simulink library "snn_champions_lib"  (R2026a)
settings: Solver=VariableStepAuto
(part 11 of 24)

== matlab function snn_champions_lib/Donatello_Tier/VS/SLOW_n8/DEC ==
  data: raw input; v0 output; valid input; T output; s0 output; a output; b output
function [v0, T, s0, a, b] = DEC(raw, valid)
%#codegen
% [SPLIT] Solo il decode: latch di raw + fasi. Riceve raw(5)+valid dalla MF SNN (entita' a se').
  persistent pv rawl dodec
  if isempty(pv)
    pv = fi(zeros(5,1), 1, 21, 13);
    rawl = fi(zeros(5,1), 1, 21, 13);
    dodec = false;
  end
  if dodec
    pv = snn_decode_lut(rawl, 64);
    dodec = false;
  end
  if valid
    rawl(:) = raw;               % latch DOPO la catena: rawl e' un vero registro
    dodec = true;
  end
  v0 = pv(1); T = pv(2); s0 = pv(3); a = pv(4); b = pv(5);
end

% ====================================================================================
% Funzioni locali INLINATE dai sorgenti veri (build_hdl_variants le legge a build-time).
% Le funzioni locali hanno precedenza sul path => il blocco e' SELF-CONTAINED.
% NON modificarle qui: si rigenerano con build_hdl_variants.
% ====================================================================================

function p = snn_decode_lut(raw, N) %#codegen
%SNN_DECODE_LUT  Decode Donatello con sigmoide via LUT a N punti su [-8,8) + interp lineare.
%  Generalizza snn_decode_hdl (N=256). N = coder.const, potenza di 2 (scala indice = N/16).
%  Costanti Donatello baked (lo sweep e' Donatello-only). Bit-identico a snn_decode_hdl per N=256.
%
%  ⚠️ SINGLE SOURCE (R4, 2026-07-19): il corpo e' ora la composizione di decode_a + decode_b, che sono
%  le DUE FASI che la chart esegue in due clock distinti -- il decode era il collo (pv_3, 31 livelli:
%  quattro moltiplicatori in serie piu' la lettura di tabella, tutto in un clock).
%  Composte qui in una chiamata sola perche' (a) i chiamanti non cambiano (snn_top_b2, le varianti
%  Donatello_LUT16..512) e (b) i cancelli provano ESATTAMENTE il codice che gira in hardware, non un
%  suo gemello. Il taglio e' fra `frac` e la lettura di `sgtab`: espressioni invariate, solo separate.
  [k, frac] = decode_a(raw, N);
  sv        = decode_b(k, frac, N);
  p         = decode_c(sv);   % [R10] scalatura finale in una fase a se'
end


function [k, frac] = decode_a(raw, N) %#codegen
%DECODE_A  [R4/R12] Prima meta' del decode: dal readout grezzo all'INDICE di tabella + frazione.
%
%  ⚠️ SINGLE SOURCE: composizione di decode_a1 (normalizzazione) e decode_a2 (scala/indice/frazione),
%  che la chart esegue in DUE clock -- i due moltiplicatori erano in serie (collo a 57,5 MHz).
%  Composta qui per i chiamanti funzionali (snn_decode_lut) e perche' i cancelli provino il codice vero.
%
%  ⚠️ NON si time-multiplexano i 5 parametri (restano srotolati): sarebbe un'ottimizzazione di AREA, e
%  di area ce n'e' in abbondanza. Serve solo profondita'.
  adjv        = decode_a1(raw);
  [k, frac]   = decode_a2(adjv, N);
end


function adjv = decode_a1(raw) %#codegen
%DECODE_A1  [R12] Prima parte del decode: normalizzazione (raw - offset)*invtau.
%  Separata da decode_a2 perche' i due moltiplicatori (invtau e scale) erano in serie nello stesso
%  clock -- era il collo a 57,5 MHz (dfrv, 18 livelli). `adj` ha il tipo Tadj GIA' DICHIARATO
%  nell'originale, quindi qui non si stringe nulla (nessun rischio §2.1).
%  Espressione VERBATIM da snn_decode_lut.
  Traw  = numerictype(1,21,13); Tadj = numerictype(1,18,13); Titau = numerictype(1,18,16);
  offset = coder.const(fi([-0.40404 -0.39012 1.7718 2.6884 -0.95578].', Traw));
  invtau = coder.const(fi([0.1 1/3 0.1 1/3 1/3].', Titau));
  adjv = fi(zeros(5,1), Tadj);
  for i = 1:5
    adjv(i) = fi((raw(i) - offset(i)) * invtau(i), Tadj);
  end
end


function [k, frac] = decode_a2(adjv, N) %#codegen
%DECODE_A2  [R12] Seconda parte: scala su [0,N), indice di tabella e frazione.
%  Espressioni VERBATIM da snn_decode_lut, con `adj` gia' calcolato da decode_a1.
  Tadj = numerictype(1,18,13); Ts = numerictype(1,16,14); Tsc = numerictype(0,23,13);
  scale = coder.const(N / 16);                                    % punti per unita' su [-8,8)
  Tsm   = numerictype(0, 8, 0);                                   % moltiplicatore scala (<=32)
  k    = zeros(5, 1, 'int32');
  frac = fi(zeros(5,1), Ts);
  for i = 1:5
    scaled = fi((adjv(i) + fi(8, Tadj)) * fi(scale, Tsm), Tsc);    % (adj+8)*scale in [0,N)
    ki = int32(floor(scaled));
    if ki < int32(0),     ki = int32(0);     end
    if ki > int32(N - 2), ki = int32(N - 2); end
    k(i)    = ki;
    frac(i) = fi(scaled - fi(double(ki), Tsc), Ts);
  end
end


function sv = decode_b(k, frac, N) %#codegen
%DECODE_B  [R4/R10/R17] Seconda fase del decode: tabella + interpolazione lineare -> s.
%  ⚠️ SINGLE SOURCE: composizione di decode_b1 (letture + differenza) e decode_b2 (interpolazione), che
%  la chart esegue in DUE clock. Composta qui per i chiamanti funzionali e per i cancelli.
  [s0v, delv] = decode_b1(k, N);
  sv          = decode_b2(s0v, delv, frac);
end


function [s0v, delv] = decode_b1(k, N) %#codegen
%DECODE_B1  [R17] Letture della tabella + differenza: s0 = sgtab(k), del = sgtab(k+1) - sgtab(k).
%  Separata da decode_b2 perche' letture, sottrazione, moltiplicazione e somma erano tutte nello stesso
%  clock -- era il collo a 77,6 MHz (dsv, 14 livelli). Espressioni VERBATIM da snn_decode_lut.
  Ts    = numerictype(1,16,14);
  scale = coder.const(N / 16);
  sgtab = coder.const(fi(1 ./ (1 + exp(-(-8 + (0:N-1) / scale))), Ts));  % 1xN
  s0v  = fi(zeros(5,1), Ts);
  delv = fi(zeros(5,1), Ts);
  for i = 1:5
    s0 = sgtab(k(i) + 1); s1 = sgtab(k(i) + 2);
    s0v(i)  = s0;
    delv(i) = fi(s1 - s0, Ts);
  end
end


function sv = decode_b2(s0v, delv, frac) %#codegen
%DECODE_B2  [R17] Interpolazione lineare: s = s0 + frac*del. Espressione VERBATIM da snn_decode_lut.
  Ts = numerictype(1,16,14);
  sv = fi(zeros(5,1), Ts);
  for i = 1:5
    sv(i) = fi(s0v(i) + frac(i) * delv(i), Ts);
  end
end


function p = decode_c(sv) %#codegen
%DECODE_C  Scalatura finale -> i 5 parametri. [R10] fase a se' nel controllore.
%  [A3] Ora e' la COMPOSIZIONE di decode_c1 (i prodotti, a precisione piena) + decode_c2 (somma
%  dell'offset + cast). Composta qui perche' (a) i chiamanti non cambiano e (b) i cancelli provano
%  ESATTAMENTE il codice che gira in hardware, non un suo gemello.
%  La chart nella variante `p6` chiama le due meta' in due fasi distinte: e' li' che il taglio serve,
%  perche' separa i DSP dalla catena di CARRY4 che domina il path critico.
  pr = decode_c1(sv);
  p  = decode_c2(pr);
end


function pr = decode_c1(sv) %#codegen
%DECODE_C1  [A3] Prima meta' di decode_c: i SOLI PRODOTTI hilo.*sv.
%  Taglio dentro l'operazione, non fra le operazioni: il collo di Donatello e' `lo + hilo*sv`, dove i
%  DSP fanno la moltiplicazione ma la somma finisce in fabric come catena di 15 CARRY4 in serie
%  (misurato: 24,307 ns = logica 15,490 + routing 8,817, 23 livelli).
%  Registrare il prodotto separa DSP e addizionatore in due clock.
%
%  ⚠️ LARGHEZZA PIENA: il prodotto NON va stretto qui. Stringere un parziale prima dell'uso e' il bug
%  §2.1 di questo progetto — cambierebbe la matematica. Il tipo si lascia DEDURRE dall'espressione.
  Tp   = numerictype(1,21,13);
  hilo = coder.const(fi([37 2 4 2.2 2.5].', Tp));
  pr   = hilo .* sv;                  % tipo dedotto = precisione piena
end


function p = decode_c2(pr) %#codegen
%DECODE_C2  [A3] Seconda meta' di decode_c: somma dell'offset + cast finale ai 5 parametri.
%  Riceve il prodotto a PRECISIONE PIENA da decode_c1 (registrato) e fa `lo + pr`, poi il cast a Q8.13.
%  Aritmetica IDENTICA a decode_c: stesso ordine, stesso singolo cast finale -> bit-exact per
%  costruzione. Ma "per costruzione" non e' un cancello: lo prova run_block_traj_test (dmax=0).
  Tp = numerictype(1,21,13);
  lo = coder.const(fi([8 0.5 1 0.3 0.5].', Tp));
  p  = fi(zeros(5,1), Tp);
  for i = 1:5
    p(i) = fi(lo(i) + pr(i), Tp);
  end
end

== matlab function snn_champions_lib/Leonardo/SNN ==
  data: x_phys input; params output
function params = SNN(x_phys)
%#codegen
% Blocco champion SELF-CONTAINED: pesi bakati + forward ALIF + decode, zero dipendenze .m.
  W_IN  = [0.25 1 0 0.5;-0.25 0.125 -1 1;0.125 -0.5 1 0.5;1 0.25 0.5 -0.25;1 0.25 -0.25 0.125;-0.25 0.5 -0.5 1;-1 -0.5 -0.5 -1;-0.0625 -1 1 -1;0.5 0.125 -0.5 0.5;-0.125 1 0.25 -0.5;-0.125 -0.125 0.5 1;0.5 -0.0625 1 0;1 -0.5 -0.5 0.5;-1 1 0.25 0.0625;0.25 -0.25 1 -1;0 -0.5 0.25 -0.125;0.5 -0.125 1 -0.5;-1 -1 0.5 0.0625;1 -0.5 -1 -0.5;-1 0.5 0.25 1;-1 -1 1 0;0.5 -0.5 0.25 -1;-0.5 0.5 0.25 -0.25;0.5 1 -0.5 -0.25;0.5 -0.25 -0.5 -1;-0.5 0.25 -0.5 -0.5;0.25 -0.5 -1 -0.25;-2 -0.5 1 0.0625;0.5 -1 -1 -1;0.125 -1 0.125 0.5;0.5 -0.5 -0.25 -0.5;-0.5 -0.25 -0.25 0.5];
  U     = [-0.25 0.0625 -0.125 -0.125 -0.25 0.0625 0.25 0.0625;-0.0625 -0.125 0.125 0.0625 -0.125 -0.0625 0 -0.0625;-0.125 -0.0625 -0.125 -0.0625 -0.0625 0 0.125 0;0.125 0.0625 0.125 0.125 -0.0625 0.0625 -0.25 0;0.125 0.0625 0.125 0.25 0.125 -0.0625 0 -0.0625;0.25 -0.125 0.25 0.25 0 -0.125 -0.25 -0.25;0.25 -0.25 0.5 0.0625 0.25 -0.25 -0.5 -0.5;0.25 -0.125 0.25 0.125 0.125 -0.125 -0.25 -0.25;0.125 -0.125 0.25 0 0.5 -0.25 -0.25 -0.125;-0.125 0.25 -0.25 0 -0.125 0.25 0.25 0.25;-0.25 0.0625 -0.25 -0.125 -0.25 0 0.25 0.125;-0.125 0.25 -0.125 -0.125 0 0.0625 0.25 0.125;0.125 0.125 0.0625 0.25 0.25 0.125 0 -0.0625;0.0625 0 0.0625 0.125 -0.25 0.125 0 0.125;-0.25 0.125 -0.0625 -0.25 0.125 0.0625 0.125 0.125;-0.125 -0.0625 -0.125 0.125 -0.25 -0.125 0.0625 0;0.5 -0.25 0.25 -0.0625 0.5 -0.5 -0.5 -0.25;0.125 -0.25 0.125 0.125 0.25 -0.25 -0.25 -0.0625;0.25 -0.25 0.25 0.0625 0.125 -0.25 -0.25 -0.25;-0.0625 -0.125 0 0.125 -0.25 0 0.125 0.0625;-0.25 0.125 -0.25 -0.125 -0.0625 0.125 0.25 0.25;0.25 -0.25 0.25 0.125 0.25 -0.25 -0.25 -0.25;0.125 -0.0625 0.0625 0.5 0.0625 0.25 0 0;0.125 -0.25 0.25 0.5 0.125 -0.125 0 -0.25;-0.25 -0.0625 -0.0625 0 -0.0625 0 0.25 0;0.5 -0.25 0.25 0.25 0.25 -0.5 -0.25 -0.25;0.5 -0.5 0.5 0.5 0.25 -0.25 -0.5 -0.5;0.125 -0.25 0.25 0.125 0.25 -0.0625 0.0625 -0.125;0.5 -0.25 0.5 0.0625 0.5 -0.5 -0.5 -0.5;-0.25 0.25 -0.5 -0.25 -0.25 0.25 0.5 0.5;0.5 -0.5 0.5 0.125 0.5 -0.5 -0.5 -0.25;0 -0.0625 0.125 -0.0625 0.0625 -0.125 -0.125 -0.0625];
  V     = [0.0625 -0.25 -0.125 0.25 0.25 0.125 0 -0.125 -0.25 0.25 -0.125 -0.0625 0 0.125 -0.125 0.0625 -0.125 -0.25 -0.25 -0.125 -0.25 -0.25 1 0.25 0.25 -0.0625 -0.0625 -0.25 0 0 -0.125 0;-0.125 -0.125 -0.0625 0 0 -0.125 0 0.125 0.5 -0.125 0 0.0625 -0.125 -0.125 -0.125 0.125 0.25 0.25 -0.25 -0.25 0 -0.25 -0.25 0 -0.25 -0.125 -0.0625 0.0625 0 0 0.125 0;0.125 0.0625 0 0.0625 0 0.5 0 0 -0.0625 0.125 0 -0.0625 0.25 0.125 0 0 -0.125 -0.25 0.25 0.125 -0.25 -0.25 0.5 0.125 0.125 -0.125 0.0625 -0.125 0 -0.0625 -0.125 0;0 -0.125 -0.125 0.0625 -0.0625 0 0.0625 -0.25 -0.25 0.25 -0.125 -0.125 0.125 0.125 -0.125 0.0625 -0.25 -0.25 -0.5 0.0625 -0.25 -0.5 1 0.125 0.0625 0 -0.125 0.0625 0 0 -0.25 0;0.0625 -0.5 0.0625 0.125 -0.0625 0 -0.0625 -0.25 -0.125 0.25 -0.0625 0.25 0.0625 0.0625 -0.25 -0.0625 0.0625 -0.25 -0.0625 -0.125 -0.25 -0.25 0.0625 0.125 0 -0.25 -0.125 -0.125 -0.0625 -0.125 0 -0.0625;-0.125 -0.125 -0.0625 -0.125 0 -0.25 0 0 0.25 0 -0.125 -0.125 0.25 -0.0625 -0.125 0 0.0625 0.25 -0.5 -0.0625 0.25 0.125 0 0.125 -0.25 0.125 -0.125 0.25 -0.0625 0.125 0.25 0;-0.25 0.0625 0.0625 -0.25 -0.25 -0.25 -0.0625 -0.0625 0.0625 -0.0625 -0.0625 -0.125 0 0.0625 -0.125 -0.0625 -0.0625 0.25 -0.25 0.125 0.25 0 -0.125 -0.0625 -0.25 0.25 -0.125 0.5 0 0.0625 0.125 0;-0.125 0.125 0 -0.125 0 -0.25 0 0.125 0.125 -0.0625 -0.0625 0 0.0625 -0.125 -0.0625 -0.0625 0 0.25 -0.5 -0.0625 0.25 0.0625 -0.5 0.0625 -0.125 0.0625 0 0.25 0 0.125 0.25 0.0625];
  DEL   = [3 5 1 2;2 4 4 4;2 4 0 4;5 0 5 5;1 2 2 2;4 1 4 2;0 4 0 1;0 1 0 1;2 2 1 3;1 2 5 2;0 5 1 2;0 5 3 1;2 0 0 4;2 2 3 4;4 4 5 0;4 5 0 2;0 4 4 3;5 5 4 2;4 5 4 2;3 0 3 1;3 2 0 4;0 4 2 0;5 4 5 2;4 4 3 3;5 3 4 5;2 2 3 1;3 3 5 3;1 3 0 3;1 0 3 2;2 3 4 4;2 4 5 0;1 2 4 0];
  BTH   = [1.5400424003601074;0.60637873411178589;1.2149713039398193;1.3223150968551636;1.5843478441238403;1.3005355596542358;1.4105348587036133;1.0825026035308838;1.3853039741516113;1.0379821062088013;1.2504197359085083;1.158677339553833;0.93588978052139282;1.1027405261993408;1.3031506538391113;1.3676879405975342;1.6325922012329102;1.5050898790359497;1.0741523504257202;1.2025256156921387;1.0485290288925171;1.5150537490844727;0.84104228019714355;0.99839270114898682;1.5752084255218506;1.2629411220550537;1.3518692255020142;0.76825004816055298;1.4178869724273682;1.114804744720459;1.1964786052703857;1.3985182046890259];
  TJ    = [0.53961282968521118;-0.065692238509654999;0.69547575712203979;0.39467334747314453;0.27812755107879639;0.36636638641357422;0.46853935718536377;0.28439891338348389;0.26325023174285889;0.12272599339485168;0.57048964500427246;0.35351014137268066;-0.00250800303183496;-0.027677660807967186;0.63428056240081787;0.40770524740219116;0.74491316080093384;0.59902232885360718;0.20256176590919495;-0.0053168567828834057;0.3602060079574585;0.55292367935180664;-0.0063420552760362625;-0.055277645587921143;0.62946045398712158;0.42266586422920227;0.35328882932662964;-0.024216080084443092;0.47340747714042664;0.37444651126861572;0.26409748196601868;0.46853935718536377];
  LD    = [8;8;8;8;8;8;8;8;8;8;8;8;8;8;8;8;8;8;8;8;8;8;8;8;8;8;8;8;8;8;8;8];
  W_OUT = [0.125 2 0 0.125 0.0625 0.5 -0.0625 0.5 0.125 -0.125 0.25 -0.25 0.125 0.5 0 1 -0.5 -0.25 0.5 1 0.25 1 -0.125 0.5 0.25 0.25 0.5 -2 -0.25 1 -0.5 0.5;-0.125 -0.25 -0.25 0.125 0.25 0.0625 0 0.25 0.25 -0.125 -0.25 0.0625 0.5 -0.25 -0.0625 0.25 0.25 0.0625 -0.125 -0.125 0 0.5 -0.25 0.0625 -0.5 -0.25 0.125 -0.5 0.125 0.25 0.0625 -0.0625;-0.5 -0.25 -0.5 -0.125 0.5 0.5 0.125 -0.5 0.125 -1 -1 -1 0.5 -0.5 -0.25 -0.25 -0.0625 0.0625 0.0625 -0.5 -1 -0.0625 -0.125 0.5 0.125 0 0.5 -0.125 0.125 -0.5 0.25 -0.125;-0.25 0.25 0.0625 -0.25 -0.125 -0.125 -0.125 0.125 -0.125 -0.5 -0.125 -0.25 0.0625 -0.5 0.25 -0.125 -0.0625 -0.25 0.25 -0.0625 0.125 0.5 -1 -0.5 -0.0625 -0.25 0 -0.5 -0.125 0.125 0.25 0.0625;-0.125 -0.5 -0.25 -0.0625 0.125 0.25 0.25 -0.125 0.5 -0.0625 -0.25 -0.0625 1 -0.25 -0.25 0.0625 0.125 -0.0625 0.5 -0.25 -0.25 0 -0.125 0.125 -0.125 0 -0.25 -0.25 0.25 -1 -0.125 0.25];
  P_LO  = [8;0.5;1;0.30000001192092896;0.5];
  P_HI  = [45;2.5;5;2.5;3];
  D_OFF = [-0.67073744535446167;-0.11699806153774261;-1.4559782743453979;-0.27981284260749817;-1.7696963548660278];
  L_TAU = [10;3;10;3;3];
  NRM   = [150;40;20;40];
  NT = 10; MAXD = 6; H = size(W_IN, 1);
  % --- normalizzazione (fisico -> [0,1]) ---
  xin = x_phys(:);
  dvc = min(max(xin(3), -NRM(3)), NRM(3));
  xn  = [xin(1)/NRM(1); xin(2)/NRM(2); (dvc + NRM(3))/(2*NRM(3)); xin(4)/NRM(4)];
  % --- stato persistente (registri del blocco) ---
  persistent Vm fat sprev Vli xbuf started
  if isempty(started)
    Vm = zeros(H,1); fat = zeros(H,1); sprev = zeros(H,1);
    Vli = zeros(5,1); xbuf = zeros(4, MAXD); started = true;
  end
  % --- NT tick SNN interni ---
  for k = 1:NT
    xbuf(:, 2:end) = xbuf(:, 1:end-1); xbuf(:, 1) = xn;
    Iin = zeros(H, 1);
    for dd = 0:MAXD-1
      mask = double(DEL == dd);
      Iin = Iin + (W_IN .* mask) * xbuf(:, dd+1);
    end
    rec = U * (V * sprev);
    Vm  = Vm - Vm ./ LD + Iin + rec;
    eth = BTH + max(fat, 0);
    s   = double(Vm >= eth);
    fat = fat - fat ./ LD + s .* max(TJ, 0);
    Vm  = Vm - s .* eth;
    sprev = s;
    Vli = Vli - Vli ./ 8 + W_OUT * s;
  end
  % --- decode -> 5 parametri fisici ---
  adj = (Vli - D_OFF) ./ L_TAU;
  params = P_LO + (P_HI - P_LO) .* (1 ./ (1 + exp(-adj)));
end

== matlab function snn_champions_lib/Donatello_Tier/VS/SLOW_n5/SNN ==
  data: s input; raw output; v input; dv input; v_l input; valid output
function [raw, valid] = SNN(s, v, dv, v_l)
%#codegen
% [SPLITPIPE] REGISTRO sugli OPERANDI del normalize (fra clamp e moltiplicazione): la
% moltiplicazione a 34 bit finisce in uno stadio suo -> rompe ingresso->normalize->go. La
% moltiplicazione e' a valle di op_reg; l'edge-trigger confronta gli OPERANDI registrati (equivale
% a confrontare xn, dato che mul e' deterministica). +1 clock di latenza. Fuori dal core.
  Tt = snn_types('fixed', 5);
  op = local_normalize_ops(s, v, dv, v_l);
  persistent op_reg op_prev started prime
  if isempty(started)
    op_reg = cast(zeros(4,1), 'like', op);  % init COSTANTE (non =op: eviterebbe il registro
    op_prev = op_reg;                        %  con un bypass combinatorio ingresso->mul->xbuf)
    started = true; prime = true;
    go = false;
  elseif prime
    prime = false;
    go = true;
  else
    go = any(op_reg ~= op_prev);
  end
  op_prev = op_reg;
  xn = local_normalize_mul(op_reg, Tt);
  [raw, valid] = snn_b2_fsm(xn, go);
  op_reg = op;
end

function xn = local_normalize(s, v, dv, v_l, T)
%LOCAL_NORMALIZE  fisico -> xn (fixed) = composizione ops+mul (bit-identica all'originale).
%  Nel deployato la normalize gira in SW float e all'HDL arriva gia' xn (HDL_PHASE §3.1).
  op = local_normalize_ops(s, v, dv, v_l);
  xn = local_normalize_mul(op, T);
end

function op = local_normalize_ops(s, v, dv, v_l)
%LOCAL_NORMALIZE_OPS  clamp del dv -> operandi [s; v; d_clamped; v_l] (pre-moltiplicazione).
  DVc = fi(20, 1, 24, 13);   % 24-13-1 = 10 bit interi: DV=20 ci sta
                                   % (con Q5.13/18bit saturerebbe a ~16 -> clamp sbagliato)
  d = dv;                          % clamp a +-DV. NB: d(:) = ... per NON cambiare il tipo di d
  if d >  DVc, d(:) =  DVc; end    %     (codegen: una variabile non puo' cambiare tipo, HDL_PHASE §9)
  if d < -DVc, d(:) = -DVc; end
  op = [s; v; d; v_l];
end

function xn = local_normalize_mul(op, T)
%LOCAL_NORMALIZE_MUL  operandi -> xn. RECIPROCI a Q?.30 (NON Q?.20): con Q?.20 xn devia di 1 LSB
%  ~1 volta su 25 step -> uno spike flippa -> params divergono. Con Q?.30 e ingressi >=20 bit
%  frazionari, xn e' IDENTICO al riferimento float (0 diff).
  invS   = fi(0.0066666666666666671, 1, 34, 30);
  invV   = fi(0.025000000000000001, 1, 34, 30);
  inv2DV = fi(0.025000000000000001, 1, 34, 30);
  invVL  = fi(0.025000000000000001, 1, 34, 30);
  DVc    = fi(20, 1, 24, 13);
  xn = cast(zeros(4,1), 'like', T.V);
  xn(1) = cast(op(1) * invS, 'like', T.V);
  xn(2) = cast(op(2) * invV, 'like', T.V);
  xn(3) = cast((op(3) + DVc) * inv2DV, 'like', T.V);
  xn(4) = cast(op(4) * invVL, 'like', T.V);
end

% ====================================================================================
% Funzioni locali INLINATE dai sorgenti veri (build_hdl_variants le legge a build-time).
% Le funzioni locali hanno precedenza sul path => il blocco e' SELF-CONTAINED.
% NON modificarle qui: si rigenerano con build_hdl_variants.
% ====================================================================================

function W = b2_rom_active() %#codegen
%B2_ROM_ACTIVE  Pesi del champion attivo (baked). GENERATO da gen_b2_rom('Donatello').
  W.fc = fi([1 1 -0.25 1;0.125 0.5 -0.0625 1;1 -1 1 0.125;1 0.125 0.5 -0.125;1 0.5 -0.0625 0.5;-0.0625 0.25 0 1;0 0.5 0.5 0.25;1 -0.25 2 -0.0625;1 0.125 -0.25 0.5;0.25 1 0.125 -0.25;0.25 -0.25 0.5 1;0.5 -0.5 0.5 0.25;1 0.25 -0.125 0.5;-1 1 0.25 0.5;1 0.5 1 -0.25;0.5 -0.25 0.5 0.0625;0.25 -0.25 1 -0.5;-0.5 -0.5 1 0.25;2 0 -0.25 0;-0.5 0.5 0.5 1;-0.125 -0.25 1 0;1 0.125 1 -0.5;-0.0625 1 0.5 0.125;1 1 -0.25 -0.125;2 0.5 0.5 -0.25;-0.125 0.5 0.25 -0.25;1 0.125 -0.0625 0.25;-0.5 -0.25 1 0.5;1 -0.125 0.125 0.5;1 -0.0625 0.5 0.25;1 0.5 1 0.125;0.125 0.25 0.5 0], 1, 16, 13);
  W.U = fi([0 0 -0.0625 -0.0625 -0.0625 0 0 0 -0.0625 0 0 0 0.0625 0 -0.125 0;-0.0625 0 -0.0625 0 0 0 0 0 0 0 -0.0625 0 0 0.0625 0 0;0.0625 -0.0625 -0.0625 0 -0.0625 -0.0625 0 0 0.0625 0 0.0625 0 0 0 0 0;0.0625 -0.0625 0 0 0 0 -0.0625 0 0 -0.0625 0.0625 -0.0625 0 -0.0625 0 -0.0625;0.0625 -0.0625 0 0 0 0 0.0625 0 0 0 0 -0.0625 0.0625 0 -0.0625 0;0 0.0625 0.0625 -0.0625 0.0625 0 0 0 0.0625 0.0625 0 0.0625 0 0 0 0;-0.0625 0.0625 0.0625 -0.0625 0 0 -0.0625 0.0625 0.0625 0.0625 0 0 -0.0625 0 0 0.0625;0 0 0.0625 0.0625 0 0 0 0 -0.0625 -0.0625 0 0 0 0 -0.0625 0;0 0 0 0 0.0625 -0.0625 0 0 -0.0625 -0.0625 -0.0625 0 0 0 0.0625 0;0 0 0 0 0.0625 0 0 0 0.0625 -0.0625 0 0.0625 0 0 0 0.0625;0 0 0 0 0 0 0 -0.0625 0 0 -0.0625 0 0 0 0 0.0625;0 0.0625 0 0.0625 0 0 0 0.0625 0 -0.0625 0 -0.0625 0.0625 0 0 0;-0.0625 0.0625 0 0 0 0 -0.0625 0 0.0625 0 -0.0625 0 0 0 0 0.125;0 0 0 0 0 0.0625 -0.0625 -0.0625 0 0.0625 0 0 0.0625 0.0625 0.0625 0;0.0625 0.0625 -0.0625 0 0 -0.0625 -0.0625 0 0 0 -0.0625 0 -0.0625 0 0 0;0.0625 0 0 0 -0.0625 -0.0625 -0.0625 0.0625 -0.0625 -0.0625 0 0.0625 0 0 0 0.0625;-0.0625 0 0 0 0.125 0.0625 -0.0625 -0.0625 0 0 0 0 -0.0625 0 -0.0625 0;0.0625 -0.0625 0 0.0625 0 -0.125 0 -0.0625 0 0 0.0625 -0.0625 0.0625 0 -0.0625 -0.0625;-0.0625 0 -0.0625 0.0625 -0.0625 0 -0.0625 0.0625 0.0625 -0.0625 0 0 -0.0625 0 0 -0.0625;0.0625 0.125 0 -0.0625 0 0 0 0 0.0625 0 0.0625 0.0625 0 0 -0.0625 0;0 -0.0625 0 0 -0.125 -0.0625 0 0.0625 -0.0625 -0.0625 0.0625 0 0.0625 -0.0625 -0.0625 -0.0625;0 0 0 0 -0.0625 0 0.0625 -0.0625 0 -0.0625 0.0625 0 0.0625 0 0 0;-0.0625 0.125 0 0 0 -0.0625 0 0 -0.0625 0.0625 0 0 0 0 0.0625 0;0 0 0 0 0 0 0 0 -0.0625 0 0.0625 0.125 0 0.0625 0 0.0625;0 -0.0625 0.0625 0 0 -0.0625 0 0 -0.0625 0 0 0.0625 0.0625 0 0 0;-0.0625 0 0 -0.125 0.0625 0.0625 0 0 0 0.0625 -0.0625 0.0625 -0.0625 0.0625 0.0625 0;0.0625 -0.0625 0 0 0 0 0.0625 0 -0.0625 0 0 0 0 0 0 0.0625;0 0 0 0.125 0 0 0 0.0625 -0.0625 0 0.0625 -0.0625 0 0.0625 0 0;0 0.0625 0.0625 0 0 0.0625 -0.0625 0 0 0.0625 0 0 -0.0625 0 0.0625 0.125;0 0.0625 0.0625 0.0625 0.0625 0.0625 0 0 0 0.0625 -0.0625 0.0625 -0.0625 0 0 0;0 0 0.0625 0 0 0.0625 -0.0625 -0.0625 0.0625 0.0625 -0.0625 0.125 0.0625 0 0 0;0 0 -0.0625 0.0625 0.0625 0 0 0.125 0 0.0625 0.0625 0.0625 0 -0.0625 0.0625 0], 1, 16, 13);
  W.Vr = fi([0 -0.125 -0.0625 -0.0625 0 0 -0.0625 -0.0625 0 -0.0625 -0.0625 0 0 0 -0.0625 -0.0625 0 0 0.0625 0 0 -0.125 0 0.0625 0 0 -0.0625 0 0 0 0 0;0.0625 0.0625 0 0 0 0 0.0625 0 0 0.0625 0.0625 0 0 0 0 0.0625 0 -0.0625 0 0.0625 0 0 0.0625 0 0.0625 0 0 0.125 -0.0625 0.125 0 0;0 0.0625 0 0.0625 0 0 -0.0625 0 0 0 0 0 0 0.0625 0 0 0.0625 0 0.0625 0 0 0.0625 0.0625 0 -0.0625 -0.0625 0 0 0 0.0625 0 0.0625;0 -0.0625 -0.0625 0 0 0 0 -0.0625 0 0 0.0625 0.0625 0 0 0 0.0625 0.0625 0 -0.0625 -0.0625 -0.0625 -0.0625 0.0625 0 0 0 0 0 0.0625 -0.0625 -0.0625 0;0 0 0.0625 0 -0.0625 0.0625 0.0625 0.0625 0 0 0.0625 0 0.0625 0.0625 0.0625 0 0.0625 0 0.0625 0 0.0625 0 0 0.0625 0.0625 0 0.125 0 0 0.0625 0.0625 0;0 0.0625 -0.125 0 0 0 0 0 0 -0.0625 -0.0625 0 0 0.0625 0.125 0.0625 0 0.0625 -0.0625 0.0625 0.0625 0 0.0625 -0.0625 0 -0.0625 0 0 0 0.0625 0 0;0 -0.0625 -0.0625 0 0 -0.0625 0 -0.0625 0 0 -0.0625 -0.0625 -0.0625 0.0625 -0.0625 0 0 -0.0625 0.0625 -0.125 -0.0625 0 -0.0625 -0.0625 -0.0625 0 0 -0.125 -0.0625 0 0 -0.0625;0 0 -0.0625 -0.0625 0.0625 0 -0.0625 0 -0.0625 0 0.0625 -0.0625 0.0625 0.0625 0.0625 0 0 0 0 -0.0625 0 -0.0625 0 0 0 0 -0.0625 -0.0625 0 0 0 0;-0.0625 0.0625 0 0.0625 0 0.0625 -0.0625 0 0.0625 0 0.0625 0 0 0.0625 0 0 0 0 0.0625 -0.0625 0.0625 0 0.0625 0 0 0.125 0.0625 0.0625 0.0625 0.0625 0 0;0.0625 0.0625 0 0.0625 0.0625 0.0625 0.0625 0.0625 0.0625 0 0.0625 0 0.0625 0.0625 0 -0.0625 0.0625 0 0.0625 0.0625 0 0.0625 0.0625 0 0.0625 0.0625 0 0 0 0 0 0;0 -0.0625 -0.0625 0 -0.0625 0 0 0 0 0 -0.0625 -0.125 -0.0625 -0.0625 0 -0.0625 -0.0625 0 0 -0.0625 -0.0625 0 0 0 0 -0.0625 0 -0.0625 0 0 -0.0625 0;0 0 0 0.0625 0 0 0.0625 0 0 0 0 0 0.0625 0 0 0.125 -0.0625 0 0.0625 0.0625 0 0 0.0625 0.0625 0 0.0625 0.0625 0 0 0 0 0;-0.0625 0 0 0 0.0625 0.0625 0 -0.0625 -0.0625 -0.0625 -0.0625 0 0 -0.0625 0 -0.0625 0 0 0 -0.0625 0 -0.0625 0 0 -0.0625 -0.0625 0 0 -0.0625 0 0.0625 0;0.0625 0 0 0.0625 0 0 0 -0.0625 0 0.0625 0 -0.0625 0 0.0625 0.0625 0 0.0625 0.0625 0 0.0625 0 0 0 0.0625 0.0625 0 0 0.125 0 0 0.0625 -0.0625;0.0625 0 0 0.0625 0 0.0625 0 0 0 0.0625 -0.0625 -0.0625 0 0.125 0 0 0 0 -0.0625 0 0.0625 0 0.0625 -0.0625 0.0625 0 0 0 0 0 0.0625 0;0 0 0 0.0625 0 0.0625 0 0.0625 0 0 0.0625 0.0625 0 0 0 0.0625 -0.0625 0 0.0625 0.0625 0.0625 0 0 0.0625 0.125 0 0 0 0 0 0.0625 0], 1, 19, 13);
  W.Wout = fi([-0.25 -0.125 -0.0625 -0.25 -0.25 0.25 0.25 -0.5 0.125 0.125 0.5 0.25 0.5 -0.125 0.25 0.25 -0.5 -0.25 0.0625 0.25 -0.25 0.0625 0 0.125 -0.25 0.25 0.25 -0.25 0 0 0.125 0.5;0.125 -0.125 0.25 -0.25 -0.125 0 -0.25 0 -0.25 0 0 0 -0.5 -0.5 0.125 0.25 -0.5 0.125 -0.25 0 0.25 0.25 -0.25 0.25 0.25 0 0.5 -0.25 -0.125 -0.25 0.0625 0.0625;0 -0.25 -0.25 0.125 -0.5 -0.0625 0 -0.125 0.125 0 0.25 -0.0625 -0.25 0.25 0.0625 -0.125 -0.25 0.125 -0.5 0.125 0.25 -0.5 -0.25 -0.25 0.25 0.25 0 0.5 -0.125 -0.5 0.125 0.125;0.5 0 0.25 0.25 0.25 -0.5 0.25 -0.25 0.5 0 -0.5 0.125 -0.0625 -0.5 -0.125 0.0625 0.25 -0.125 0.25 0.0625 0 0.0625 -0.25 -0.25 -0.125 -0.5 -0.25 0 -0.25 -0.125 -0.0625 -0.0625;-0.25 0 -0.0625 0.0625 0 -0.25 -0.125 -0.0625 -0.25 0 -0.0625 0.125 0.0625 0.25 -0.0625 -0.25 0.125 -0.25 -0.0625 -0.125 -0.25 -0.125 0.25 0.25 0.0625 0.25 -0.5 0.0625 0.25 0.25 -0.25 0.125], 1, 16, 13);
  W.bth = fi([1.4830578565597534;1.4914478063583374;1.4758200645446777;1.4738426208496094;1.4738566875457764;1.5251744985580444;1.5266332626342773;1.4767427444458008;1.4758551120758057;1.5250141620635986;1.5258395671844482;1.5129754543304443;1.5257152318954468;1.5249043703079224;1.5155367851257324;1.5183815956115723;1.5177655220031738;1.4894863367080688;1.4749715328216553;1.5253423452377319;1.4770052433013916;1.4827579259872437;1.5239431858062744;1.5230189561843872;1.4776254892349243;1.5125672817230225;1.5243701934814453;1.4934873580932617;1.5239229202270508;1.5202276706695557;1.5248651504516602;1.5149734020233154], 1, 19, 13);
  W.tj = fi([0.49987733364105225;0.49987733364105225;0.49987733364105225;0.49987733364105225;0.49987733364105225;0.49987733364105225;0.49987733364105225;0.49987733364105225;0.49987733364105225;0.49987733364105225;0.49987733364105225;0.49987733364105225;0.49987733364105225;0.49987733364105225;0.49987733364105225;0.49987733364105225;0.49987733364105225;0.49987733364105225;0.49987733364105225;0.49987733364105225;0.49987733364105225;0.49987733364105225;0.49987733364105225;0.49987733364105225;0.49987733364105225;0.49987733364105225;0.49987733364105225;0.49987733364105225;0.49987733364105225;0.49987733364105225;0.49987733364105225;0.49987733364105225], 1, 19, 13);
  W.delays = [3 5 1 2;2 4 4 4;2 4 0 4;5 0 5 5;1 2 2 2;4 1 4 2;0 4 0 1;0 1 0 1;2 2 1 3;1 2 5 2;0 5 1 2;0 5 3 1;2 0 0 4;2 2 3 4;4 4 5 0;4 5 0 2;0 4 4 3;5 5 4 2;4 5 4 2;3 0 3 1;3 2 0 4;0 4 2 0;5 4 5 2;4 4 3 3;5 3 4 5;2 2 3 1;3 3 5 3;1 3 0 3;1 0 3 2;2 3 4 4;2 4 5 0;1 2 4 0];
  W.sh = 3;
  W.invS = fi(0.0066666666666666671, 1, 24, 20);
  W.invV = fi(0.025000000000000001, 1, 24, 20);
  W.invVL = fi(0.025000000000000001, 1, 24, 20);
  W.inv2DV = fi(0.025000000000000001, 1, 24, 20);
  W.DV = fi(20, 1, 20, 13);
end


function T = snn_types(dt, nfrac)
%SNN_TYPES Prototipi di tipo per il core type-parametrizzato.
%  dt = 'double' (parita' vs golden) | 'fixed' (HDL, Qm.n).
%  nfrac (opz., default 5) = bit frazionari del path fixed; i bit INTERI restano
%  fissi (range invariato), varia solo la risoluzione -> per tarare i word-length
%  col ginocchio errore/risorse (run_fixed_sweep). nfrac=5 == config storica.
  if nargin < 2, nfrac = 5; end
  switch dt
    case 'double'
      z = double([]);
      T = struct('V', z, 'fatigue', z, 'acc', z, 'accw', z, 'raw', z, 'w', z);
    case 'fixed'
      f = nfrac;
      T = struct( ...
        'V',       fi([], true, 6 + f, f), ...    % Q5.f  (int 5)
        'fatigue', fi([], true, 4 + f, f), ...    % Q3.f  (int 3)
        'acc',     fi([], true, 6 + f, f), ...    % accumulatore I_input Q5.f (int 5: un tap di delay arriva a ~8)
        'accw',    fi([], true, 13 + f, f + 4), ...% accumulatore LARGO Q8.(f+4): +4 frac per shift po2 esatti
        'raw',     fi([], true, 8 + f, f), ...    % readout LI Q7.f (int 7)
        'w',       fi([], true, 3 + f, f));       % pesi po2 Q2.f (esatti per f>=5)
    otherwise
      error('snn_types:dt', 'dt deve essere ''double'' o ''fixed''');
  end
end


function [raw, valid] = snn_b2_fsm(xn, start) %#codegen
%SNN_B2_FSM  [B2] SNN Donatello time-multiplexato (1 neurone/clock) con hdl.RAM.
%  Mirror BIT-EXACT dell'aritmetica di snn_core, serializzato: V/fatigue in hdl.RAM,
%  pesi in ROM (coder.const), pipeline a 2 stadi per la latenza RAM (read->compute->write,
%  1 sola chiamata RAM/ciclo). Streaming: start=1 -> nuova control-step; valid=1 -> raw pronto.
  W = coder.const(b2_rom_active());
  T = snn_types('fixed', 5);
  hidden = 32; nt = 10; rnk = coder.const(size(W.U, 2)); out = 5; sh = W.sh;

  persistent Vram fatram xbuf xnreg t_lr t_lr_nxt V_LI wacc ...
             tickc rc written phase ...
             pR_valid pR_idx pC_valid pC_idx pC_V pC_fat rawreg inited
  if isempty(inited)
    Vram   = hdl.RAM('RAMType', 'Dual port');
    fatram = hdl.RAM('RAMType', 'Dual port');
    xbuf   = cast(zeros(4, 6), 'like', T.V);
    xnreg  = cast(zeros(4, 1), 'like', T.V);
    t_lr     = cast(zeros(rnk, 1), 'like', T.acc);
    t_lr_nxt = cast(zeros(rnk, 1), 'like', T.acc);
    V_LI = cast(zeros(out, 1), 'like', T.raw);
    wacc = cast(zeros(out, 1), 'like', T.raw);
    tickc = uint8(0); rc = uint8(0); written = uint8(0); phase = uint8(0);
    pR_valid = false; pR_idx = uint8(0);
    pC_valid = false; pC_idx = uint8(0);
    pC_V = cast(0, 'like', T.V); pC_fat = cast(0, 'like', T.fatigue);
    rawreg = cast(zeros(out, 1), 'like', T.raw);
    inited = true;
  end

  valid = false;
  raw = rawreg;

  % ---------- helper x_buf: shift + inserimento xnreg (inizio tick) ----------
  % (fatto inline dove serve)

  if phase == uint8(0)
    % IDLE: su start latcha xn, fa lo shift del tick 0, avvia la pipeline
    if start
      xnreg = xn;
      xbuf(:, 2:6) = xbuf(:, 1:5); xbuf(:, 1) = xnreg;   % tick 0 shift+insert
      tickc = uint8(0); rc = uint8(0); written = uint8(0);
      wacc = cast(zeros(out, 1), 'like', T.raw);
      pR_valid = false; pC_valid = false;
      phase = uint8(1);
    end
    % passo RAM idle (mantiene coerenza)
    [~, ~] = Vram(cast(0,'like',T.V), uint8(0), false, uint8(0));
    [~, ~] = fatram(cast(0,'like',T.fatigue), uint8(0), false, uint8(0));
    return;
  end

  % ---------- FASE 1: RUN (pipeline 2-stadi, 1 chiamata RAM/ciclo) ----------
  % indirizzo di lettura per questo ciclo (neurone rc, se ancora da leggere)
  if rc < uint8(hidden), rdAddr = rc; else, rdAddr = uint8(0); end

  % UNA chiamata RAM: scrive il risultato dello stadio C (pC), legge rdAddr
  [~, Vread]   = Vram(pC_V,   pC_idx, pC_valid, rdAddr);
  [~, fatread] = fatram(pC_fat, pC_idx, pC_valid, rdAddr);
  if pC_valid
    written = written + uint8(1);
  end

  % --- STADIO C (compute): calcola il neurone i cui dati arrivano ORA (pR) ---
  nC_valid = false; nC_idx = uint8(0);
  nC_V = cast(0, 'like', T.V); nC_fat = cast(0, 'like', T.fatigue);
  if pR_valid
    i = double(pR_idx) + 1;
    Ii = cast(0, 'like', T.accw);
    for j = 1:4
      col = double(W.delays(i, j)) + 1;
      Ii(:) = Ii + cast(cast(W.fc(i, j), 'like', T.w) * xbuf(j, col), 'like', T.accw);
    end
    % [2d R2] accumulo reci ad ALBERO bilanciato (profondita' rnk->log2(rnk)) invece del ripple
    % sequenziale: taglia il path critico. Bit-exact SE gli intermedi non saturano T.accw (verificato
    % dal parity 0/60000; il ripple originale non satura sul dataset -> ribilanciare l'ordine e' esatto).
    % Loop a bound FISSO (lvsz coder.const) -> HDL Coder li srotola come i for gia' presenti; rnk in {8,16}.
    reci_p = cast(zeros(rnk, 1), 'like', T.accw);
    for r = 1:rnk
      reci_p(r) = cast(cast(W.U(i, r), 'like', T.w) * t_lr(r), 'like', T.accw);
    end
    lvsz = coder.const(round(rnk ./ 2 .^ (1:log2(rnk))));   % rnk=16 -> [8 4 2 1]
    for lev = 1:numel(lvsz)
      for q = 1:lvsz(lev)
        reci_p(q) = cast(reci_p(2*q - 1) + reci_p(2*q), 'like', T.accw);
      end
    end
    reci = reci_p(1);
    % (Ii+reci) RESTA in T.accw (Q8.17): il cast a T.V (Q5.13) buttava i 4 bit frazionari extra
    % di accw PRIMA del confronto di soglia -> spike decisi diversamente da snn_core quando Vi cade
    % entro ~2^-14 da eth (misurato: 82,4% dei control-step del dataset divergenti). Vedi HDL_PHASE §2.1.
    % Come snn_core.m:64  ->  Vi = leaky(V(i), sh) + (Ii + reci);
    Vi  = cast(Vread - bitsra(Vread, sh), 'like', T.V) + (Ii + reci);
    eth = cast(W.bth(i), 'like', T.V) + cast(max(fatread, cast(0,'like',T.fatigue)), 'like', T.V);
    si  = Vi >= eth;
    sib = cast(si, 'like', T.V);
    nC_fat   = cast(cast(fatread - bitsra(fatread, sh), 'like', T.fatigue) + sib * cast(W.tj(i), 'like', T.V), 'like', T.fatigue);
    nC_V     = cast(Vi - sib * eth, 'like', T.V);
    nC_valid = true; nC_idx = pR_idx;
    if si
      for o = 1:out
        wacc(o) = cast(wacc(o) + W.Wout(o, i), 'like', T.raw);
      end
      for r = 1:rnk
        t_lr_nxt(r) = cast(t_lr_nxt(r) + cast(W.Vr(r, i), 'like', T.acc), 'like', T.acc);
      end
    end
  end

  % --- STADIO R (read schedule): programma la lettura del neurone rc ---
  nR_valid = false; nR_idx = uint8(0);
  if rc < uint8(hidden)
    nR_valid = true; nR_idx = rc;
    rc = rc + uint8(1);
  end

  % avanza i registri pipeline
  pR_valid = nR_valid; pR_idx = nR_idx;
  pC_valid = nC_valid; pC_idx = nC_idx; pC_V = nC_V; pC_fat = nC_fat;

  % --- fine tick: tutti i 32 neuroni scritti ---
  if written >= uint8(hidden)
    V_LI = cast(cast(V_LI - bitsra(V_LI, 3), 'like', T.raw) + wacc, 'like', T.raw);
    wacc = cast(zeros(out, 1), 'like', T.raw);
    t_lr = t_lr_nxt;
    t_lr_nxt = cast(zeros(rnk, 1), 'like', T.acc);
    written = uint8(0); rc = uint8(0);
    pR_valid = false; pC_valid = false;
    if tickc >= uint8(nt - 1)
      rawreg = V_LI; raw = V_LI; valid = true;
      phase = uint8(0); tickc = uint8(0);
    else
      tickc = tickc + uint8(1);
      xbuf(:, 2:6) = xbuf(:, 1:5); xbuf(:, 1) = xnreg;   % shift+insert per il tick successivo
    end
  end
end

% ---- ROM pesi del champion attivo: in b2_rom_active.m (baked, GENERATO da gen_b2_rom(name)) ----

== matlab function snn_champions_lib/Donatello_Tier/VS/SLOW_n5/DEC ==
  data: raw input; v0 output; valid input; T output; s0 output; a output; b output
function [v0, T, s0, a, b] = DEC(raw, valid)
%#codegen
% [SPLIT] Solo il decode: latch di raw + fasi. Riceve raw(5)+valid dalla MF SNN (entita' a se').
  persistent pv rawl dodec
  if isempty(pv)
    pv = fi(zeros(5,1), 1, 21, 13);
    rawl = fi(zeros(5,1), 1, 21, 13);
    dodec = false;
  end
  if dodec
    pv = snn_decode_lut(rawl, 64);
    dodec = false;
  end
  if valid
    rawl(:) = raw;               % latch DOPO la catena: rawl e' un vero registro
    dodec = true;
  end
  v0 = pv(1); T = pv(2); s0 = pv(3); a = pv(4); b = pv(5);
end

% ====================================================================================
% Funzioni locali INLINATE dai sorgenti veri (build_hdl_variants le legge a build-time).
% Le funzioni locali hanno precedenza sul path => il blocco e' SELF-CONTAINED.
% NON modificarle qui: si rigenerano con build_hdl_variants.
% ====================================================================================

function p = snn_decode_lut(raw, N) %#codegen
%SNN_DECODE_LUT  Decode Donatello con sigmoide via LUT a N punti su [-8,8) + interp lineare.
%  Generalizza snn_decode_hdl (N=256). N = coder.const, potenza di 2 (scala indice = N/16).
%  Costanti Donatello baked (lo sweep e' Donatello-only). Bit-identico a snn_decode_hdl per N=256.
%
%  ⚠️ SINGLE SOURCE (R4, 2026-07-19): il corpo e' ora la composizione di decode_a + decode_b, che sono
%  le DUE FASI che la chart esegue in due clock distinti -- il decode era il collo (pv_3, 31 livelli:
%  quattro moltiplicatori in serie piu' la lettura di tabella, tutto in un clock).
%  Composte qui in una chiamata sola perche' (a) i chiamanti non cambiano (snn_top_b2, le varianti
%  Donatello_LUT16..512) e (b) i cancelli provano ESATTAMENTE il codice che gira in hardware, non un
%  suo gemello. Il taglio e' fra `frac` e la lettura di `sgtab`: espressioni invariate, solo separate.
  [k, frac] = decode_a(raw, N);
  sv        = decode_b(k, frac, N);
  p         = decode_c(sv);   % [R10] scalatura finale in una fase a se'
end


function [k, frac] = decode_a(raw, N) %#codegen
%DECODE_A  [R4/R12] Prima meta' del decode: dal readout grezzo all'INDICE di tabella + frazione.
%
%  ⚠️ SINGLE SOURCE: composizione di decode_a1 (normalizzazione) e decode_a2 (scala/indice/frazione),
%  che la chart esegue in DUE clock -- i due moltiplicatori erano in serie (collo a 57,5 MHz).
%  Composta qui per i chiamanti funzionali (snn_decode_lut) e perche' i cancelli provino il codice vero.
%
%  ⚠️ NON si time-multiplexano i 5 parametri (restano srotolati): sarebbe un'ottimizzazione di AREA, e
%  di area ce n'e' in abbondanza. Serve solo profondita'.
  adjv        = decode_a1(raw);
  [k, frac]   = decode_a2(adjv, N);
end


function adjv = decode_a1(raw) %#codegen
%DECODE_A1  [R12] Prima parte del decode: normalizzazione (raw - offset)*invtau.
%  Separata da decode_a2 perche' i due moltiplicatori (invtau e scale) erano in serie nello stesso
%  clock -- era il collo a 57,5 MHz (dfrv, 18 livelli). `adj` ha il tipo Tadj GIA' DICHIARATO
%  nell'originale, quindi qui non si stringe nulla (nessun rischio §2.1).
%  Espressione VERBATIM da snn_decode_lut.
  Traw  = numerictype(1,21,13); Tadj = numerictype(1,18,13); Titau = numerictype(1,18,16);
  offset = coder.const(fi([-0.40404 -0.39012 1.7718 2.6884 -0.95578].', Traw));
  invtau = coder.const(fi([0.1 1/3 0.1 1/3 1/3].', Titau));
  adjv = fi(zeros(5,1), Tadj);
  for i = 1:5
    adjv(i) = fi((raw(i) - offset(i)) * invtau(i), Tadj);
  end
end


function [k, frac] = decode_a2(adjv, N) %#codegen
%DECODE_A2  [R12] Seconda parte: scala su [0,N), indice di tabella e frazione.
%  Espressioni VERBATIM da snn_decode_lut, con `adj` gia' calcolato da decode_a1.
  Tadj = numerictype(1,18,13); Ts = numerictype(1,16,14); Tsc = numerictype(0,23,13);
  scale = coder.const(N / 16);                                    % punti per unita' su [-8,8)
  Tsm   = numerictype(0, 8, 0);                                   % moltiplicatore scala (<=32)
  k    = zeros(5, 1, 'int32');
  frac = fi(zeros(5,1), Ts);
  for i = 1:5
    scaled = fi((adjv(i) + fi(8, Tadj)) * fi(scale, Tsm), Tsc);    % (adj+8)*scale in [0,N)
    ki = int32(floor(scaled));
    if ki < int32(0),     ki = int32(0);     end
    if ki > int32(N - 2), ki = int32(N - 2); end
    k(i)    = ki;
    frac(i) = fi(scaled - fi(double(ki), Tsc), Ts);
  end
end


function sv = decode_b(k, frac, N) %#codegen
%DECODE_B  [R4/R10/R17] Seconda fase del decode: tabella + interpolazione lineare -> s.
%  ⚠️ SINGLE SOURCE: composizione di decode_b1 (letture + differenza) e decode_b2 (interpolazione), che
%  la chart esegue in DUE clock. Composta qui per i chiamanti funzionali e per i cancelli.
  [s0v, delv] = decode_b1(k, N);
  sv          = decode_b2(s0v, delv, frac);
end


function [s0v, delv] = decode_b1(k, N) %#codegen
%DECODE_B1  [R17] Letture della tabella + differenza: s0 = sgtab(k), del = sgtab(k+1) - sgtab(k).
%  Separata da decode_b2 perche' letture, sottrazione, moltiplicazione e somma erano tutte nello stesso
%  clock -- era il collo a 77,6 MHz (dsv, 14 livelli). Espressioni VERBATIM da snn_decode_lut.
  Ts    = numerictype(1,16,14);
  scale = coder.const(N / 16);
  sgtab = coder.const(fi(1 ./ (1 + exp(-(-8 + (0:N-1) / scale))), Ts));  % 1xN
  s0v  = fi(zeros(5,1), Ts);
  delv = fi(zeros(5,1), Ts);
  for i = 1:5
    s0 = sgtab(k(i) + 1); s1 = sgtab(k(i) + 2);
    s0v(i)  = s0;
    delv(i) = fi(s1 - s0, Ts);
  end
end


function sv = decode_b2(s0v, delv, frac) %#codegen
%DECODE_B2  [R17] Interpolazione lineare: s = s0 + frac*del. Espressione VERBATIM da snn_decode_lut.
  Ts = numerictype(1,16,14);
  sv = fi(zeros(5,1), Ts);
  for i = 1:5
    sv(i) = fi(s0v(i) + frac(i) * delv(i), Ts);
  end
end


function p = decode_c(sv) %#codegen
%DECODE_C  Scalatura finale -> i 5 parametri. [R10] fase a se' nel controllore.
%  [A3] Ora e' la COMPOSIZIONE di decode_c1 (i prodotti, a precisione piena) + decode_c2 (somma
%  dell'offset + cast). Composta qui perche' (a) i chiamanti non cambiano e (b) i cancelli provano
%  ESATTAMENTE il codice che gira in hardware, non un suo gemello.
%  La chart nella variante `p6` chiama le due meta' in due fasi distinte: e' li' che il taglio serve,
%  perche' separa i DSP dalla catena di CARRY4 che domina il path critico.
  pr = decode_c1(sv);
  p  = decode_c2(pr);
end


function pr = decode_c1(sv) %#codegen
%DECODE_C1  [A3] Prima meta' di decode_c: i SOLI PRODOTTI hilo.*sv.
%  Taglio dentro l'operazione, non fra le operazioni: il collo di Donatello e' `lo + hilo*sv`, dove i
%  DSP fanno la moltiplicazione ma la somma finisce in fabric come catena di 15 CARRY4 in serie
%  (misurato: 24,307 ns = logica 15,490 + routing 8,817, 23 livelli).
%  Registrare il prodotto separa DSP e addizionatore in due clock.
%
%  ⚠️ LARGHEZZA PIENA: il prodotto NON va stretto qui. Stringere un parziale prima dell'uso e' il bug
%  §2.1 di questo progetto — cambierebbe la matematica. Il tipo si lascia DEDURRE dall'espressione.
  Tp   = numerictype(1,21,13);
  hilo = coder.const(fi([37 2 4 2.2 2.5].', Tp));
  pr   = hilo .* sv;                  % tipo dedotto = precisione piena
end


function p = decode_c2(pr) %#codegen
%DECODE_C2  [A3] Seconda meta' di decode_c: somma dell'offset + cast finale ai 5 parametri.
%  Riceve il prodotto a PRECISIONE PIENA da decode_c1 (registrato) e fa `lo + pr`, poi il cast a Q8.13.
%  Aritmetica IDENTICA a decode_c: stesso ordine, stesso singolo cast finale -> bit-exact per
%  costruzione. Ma "per costruzione" non e' un cancello: lo prova run_block_traj_test (dmax=0).
  Tp = numerictype(1,21,13);
  lo = coder.const(fi([8 0.5 1 0.3 0.5].', Tp));
  p  = fi(zeros(5,1), Tp);
  for i = 1:5
    p(i) = fi(lo(i) + pr(i), Tp);
  end
end
